simulink model "NonLinPureAnn"  (R2017a)
settings: Solver=ode45  StartTime=0.0  StopTime=400  RelTol=1e-3  EnableMultiTasking=on
libraries: simulink x2, ann x2
settings Model: Creator=Raj  LastModifiedBy=Jaydeep
settings DataIOCC: LimitDataPoints=on  SaveFormat=Array
settings OptimizationCC: LifeSpan=inf
settings DebuggingCC: UnderspecifiedInitializationDetection=Classic  MergeDetectMultiDrivingBlocksExec=none  SolverPrmCheckMsg=warning  StateNameClashWarn=warning  SFUnexpectedBacktrackingDiag=warning  SFNoUnconditionalDefaultTransitionDiag=warning  SFExecutionAtInitializationDiag=none
settings HardwareCC: ProdBitPerPointer=32  ProdBitPerSizeT=32  ProdBitPerPtrDiffT=32  ProdLargestAtomicFloat=None  ProdIntDivRoundTo=Undefined  ProdEndianess=Unspecified  ProdWordSize=32  ProdHWDeviceType=32-bit Generic
settings ModelReferenceCC: PropagateSignalLabelsOutOfModel=off
settings GRTTargetCC: TargetLangStandard=C89/C90 (ANSI)  GeneratePreprocessorConditionals=Disable all
settings ConfigComp: CovMetricSettings=dw  CovHtmlReporting=on  CovSaveCumulativeToWorkspaceVar=on  CovSaveSingleToWorkspaceVar=on  CovExternalEMLEnable=off

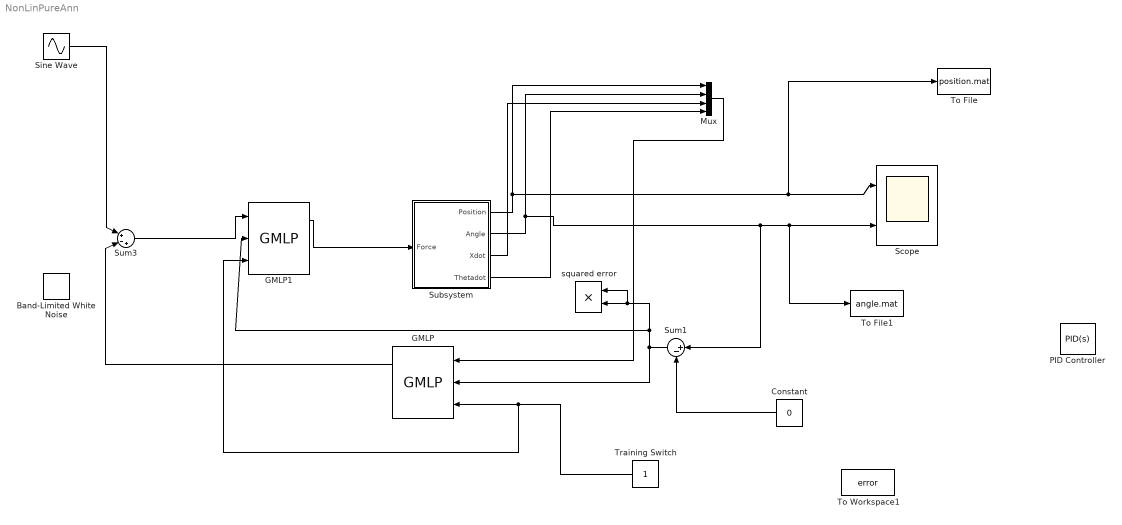
== system NonLinPureAnn ==
  Band-Limited White Noise : simulink/Sources/Band-Limited White Noise  Cov=[0.1]  Ts=0.1  seed=[23341]
  Constant : Constant  Value=0
  GMLP : ann/GMLP  dim=[4 100 100 1]  eta=[0.003 0.003 0.003 0.003]  L=[inf inf inf inf]  alp=0.01  ini=0.01  T=0.05
  GMLP1 : ann/GMLP  dim=[100 101 100 1]  eta=[0.03 0.03 0.003 0.03]/10  L=[inf inf inf inf]  alp=0.01  ini=0.01  T=0.05
  Mux : Mux
  PID Controller : simulink/Continuous/PID Controller  Controller=PID  TimeDomain=Continuous-time  SampleTime=-1  IntegratorMethod=Forward Euler  FilterMethod=Forward Euler  Form=Parallel  UseFilter=on  ControllerParametersSource=internal  P=46.1984664041102  I=10.7409360427114  D=5.8397835981222  N=99.9332249108799  InitialConditionSource=internal  InitialConditionForIntegrator=0  InitialConditionForFilter=0  ExternalReset=none  LimitOutput=off  UpperSaturationLimit=inf  LowerSaturationLimit=-inf  LinearizeAsGain=on  AntiWindupMode=none  Kb=1  TrackingMode=off  Kt=1  PParamMin=[]  PParamMax=[]  IParamMin=[]  IParamMax=[]  DParamMin=[]  DParamMax=[]  NParamMin=[]  NParamMax=[]  KbParamMin=[]  KbParamMax=[]  KtParamMin=[]  KtParamMax=[]  POutMin=[]  POutMax=[]  IOutMin=[]  IOutMax=[]  DOutMin=[]  DOutMax=[]  NOutMin=[]  NOutMax=[]  KbOutMin=[]  KbOutMax=[]  KtOutMin=[]  KtOutMax=[]  IntegratorOutMin=[]  IntegratorOutMax=[]  FilterOutMin=[]  FilterOutMax=[]  SumOutMin=[]  SumOutMax=[]  SumI1OutMin=[]  SumI1OutMax=[]  SumI2OutMin=[]  SumI2OutMax=[]  SumI3OutMin=[]  SumI3OutMax=[]  SumDOutMin=[]  SumDOutMax=[]  SaturationOutMin=[]  SaturationOutMax=[]  IntegratorContinuousStateAttributes=''  IntegratorStateMustResolveToSignalObject=off  IntegratorRTWStateStorageClass=Auto  FilterContinuousStateAttributes=''  FilterStateMustResolveToSignalObject=off  FilterRTWStateStorageClass=Auto  DifferentiatorICPrevScaledInput=0  DifferentiatorOutMin=[]  DifferentiatorOutMax=[]  InitialConditionSetting=State (most efficient)
  Scope : Scope  NumInputPorts=2
  Sine Wave : Sin  SampleTime=0
  Subsystem : Subsystem
  Sum1 : Sum  Inputs=|+-
  Sum3 : Sum  Inputs=|+-+
  To File : ToFile  Filename=position.mat  MatrixName=position
  To File1 : ToFile  Filename=angle.mat  MatrixName=angle
  To Workspace1 : ToWorkspace  VariableName=error  SaveFormat=Timeseries  SampleTime=-1
  Training Switch : Constant
  squared error : Product
  wires:
  Constant/1 -> Sum1/2
  GMLP/1 -> Sum3/2
  Training Switch/1 -> GMLP1/3, GMLP/3
  Subsystem/2(Angle) -> Mux/2, Sum1/1, To File1/1, Scope/2
  Subsystem/1(Position) -> Mux/1, To File/1, Scope/1
  Subsystem/4(Thetadot) -> Mux/4
  Subsystem/3(Xdot) -> Mux/3
  Mux/1 -> GMLP/1
  Sum1/1 -> GMLP/2, squared error/1, squared error/2, GMLP1/2
  GMLP1/1 -> Subsystem/1(Force)
  Sum3/1 -> GMLP1/1
  Sine Wave/1 -> Sum3/1

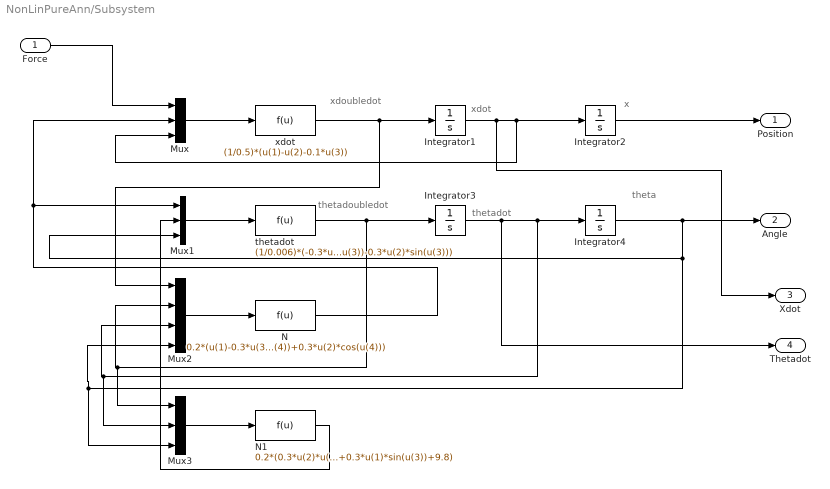
== system NonLinPureAnn/Subsystem ==
  note: xdoubledot
  note: thetadoubledot
  note: theta
  note: thetadot
  note: x
  note: xdot
  Force : Inport
  Integrator1 : Integrator  ContinuousStateAttributes='xdot'
  Integrator2 : Integrator  ContinuousStateAttributes='x'
  Integrator3 : Integrator  ContinuousStateAttributes='thetadot'
  Integrator4 : Integrator  ContinuousStateAttributes='theta'
  Mux : Mux  Inputs=3
  Mux1 : Mux  Inputs=3
  Mux2 : Mux
  Mux3 : Mux  Inputs=3
  N : Fcn  Expr=0.2*(u(1)-0.3*u(3)*u(3)*sin(u(4))+0.3*u(2)*cos(u(4)))
  N1 : Fcn  Expr=0.2*(0.3*u(2)*u(2)*cos(u(3))+0.3*u(1)*sin(u(3))+9.8)
  thetadot : Fcn  Expr=(1/0.006)*(-0.3*u(1)*cos(u(3))-0.3*u(2)*sin(u(3)))
  xdot : Fcn  Expr=(1/0.5)*(u(1)-u(2)-0.1*u(3))
  Position : Outport
  Angle : Outport  Port=2
  Xdot : Outport  Port=3  OutDataTypeStr=double
  Thetadot : Outport  Port=4
  wires:
  Integrator1/1 -> Xdot/1, Mux/3, Integrator2/1
  xdot/1 -> Mux2/1, Integrator1/1
  Mux2/1 -> N/1
  Integrator4/1 -> Angle/1, Mux2/4, Mux3/3, Mux1/3
  Integrator3/1 -> Thetadot/1, Mux3/2, Mux2/3, Integrator4/1
  thetadot/1 -> Mux3/1, Mux2/2, Integrator3/1
  Integrator2/1 -> Position/1
  Mux1/1 -> thetadot/1
  Mux/1 -> xdot/1
  N/1 -> Mux1/1, Mux/2
  Force/1 -> Mux/1
  N1/1 -> Mux1/2
  Mux3/1 -> N1/1
